simulink model "today2Proporcional"  (R2016a)
settings: Solver=VariableStepAuto  StartTime=0.0  StopTime=10.0  RelTol=1e-3
settings Model: Creator=Ivan Varabei  LastModifiedBy=Ivan Varabei

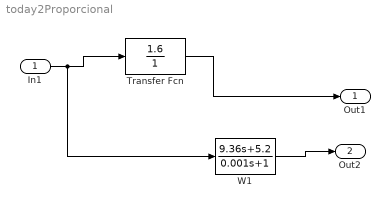
== system today2Proporcional ==
  In1 : Inport
  Transfer Fcn : TransferFcn  Numerator=[1.6]  Denominator=[1]
  "W1 " : TransferFcn  Numerator=[9.36 5.2]  Denominator=[0.001 1]
  Out1 : Outport
  Out2 : Outport  Port=2
  wires:
  Transfer Fcn/1 -> Out1/1
  In1/1 -> "W1 "/1, Transfer Fcn/1
  "W1 "/1 -> Out2/1
